simulink model "Sanepa_overall_model_Fault"  (R2023a)
settings: Solver=VariableStepAuto  StartTime=0.0  StopTime=5  RelTol=1e-3
undefined symbols (not defined in the file): D11, Delta
libraries: spsLoadFlowBusLib x44, spsThreePhaseTransformerTwoWindingsLib x23, spsThreePhaseParallelRLCLoadLib x23, spsThreePhasePISectionLineLib x18, spsThreePhaseVIMeasurementLib x4, spsThreePhaseFaultLib x4, spsThreePhaseSeriesRLCBranchLib x2, spspowerguiLib x1, spsThreePhaseSourceLib x1
settings Model: Creator=Isha Tiwari  LastModifiedBy=Dell
settings SolverCC: AlgebraicLoopSolver=TrustRegion
settings DataIOCC: SaveOutput=off  ReturnWorkspaceOutputs=off

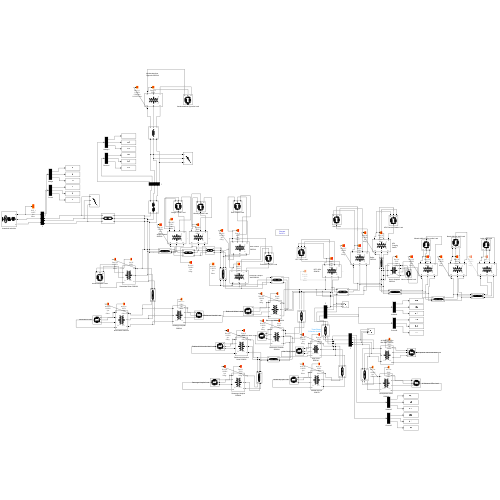
[thumbnail: Simulink's stored preview of the top-level diagram]
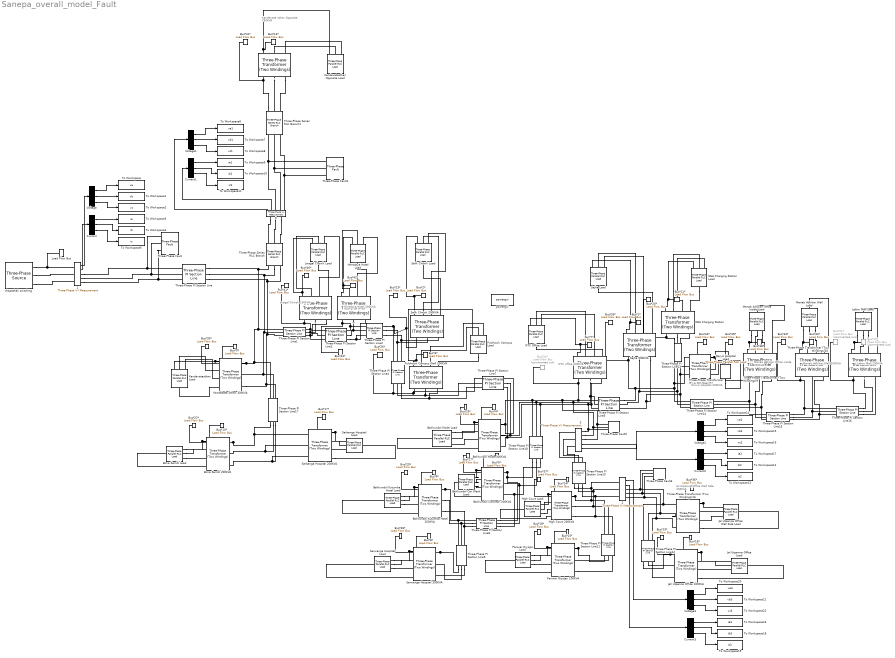
== system Sanepa_overall_model_Fault ==
  note: Norvic Hospital
      | 200KVA
  note: NTC office
      | 200KVA
  note: Manab Adhikar
      | Office inside
      | 200KVA
  note: Labim Mall
      | 200KVA
  note: Jal Utpanna Office
      | Wall Side 200KVA
  note: Manab Adhikar
      | Wall 200KVA
  note: Jwagal Chwok
      | 100KVA
  note: Himalaya Hotel
      | 300KVA
  note: Kandevata sthan
      | Opposite 250KVA
  . : spsThreePhaseTransformerTwoWindingsLib/Three-Phase Transformer (Two Windings)  Winding1Connection=Yg  Winding2Connection=Yg  CoreType=Three-limb core (core-type)  SetSaturation=off  Hysteresis=off  DataFile='hysteresis'  SetInitialFlux=off  Measurements=None  UNITS=pu  NominalPower=[ 500000 , 50 ]  Winding1=[11e3 , 0.002 , 0.08 ]  Winding2=[ 0.23e3 , 0.002 , 0.08 ]  Rm=500  Lm=500  L0=0.5  Saturation=[ 0,0 ; 0.0024,1.2 ; 1.0,1.52 ]  InitialFluxes=[ 0.8 , -0.8 , 0.7 ]  BreakLoop=off  DiscreteSolver=Trapezoidal iterative  DataType=off  TransfoNumber=1
  .. : spsThreePhaseTransformerTwoWindingsLib/Three-Phase Transformer (Two Windings)  Winding1Connection=Delta (D11)  Winding2Connection=Yn  CoreType=Three single-phase transformers  SetSaturation=off  Hysteresis=off  DataFile='hysteresis'  SetInitialFlux=off  Measurements=None  UNITS=pu  NominalPower=[ 200000 , 50 ]  Winding1=[ 11e3 , 0.002 , 0.08 ]  Winding2=[ 0.23e3 , 0.002 , 0.08 ]  Rm=500  Lm=500  L0=0.5  Saturation=[ 0,0 ; 0.0024,1.2 ; 1.0,1.52 ]  InitialFluxes=[ 0.8 , -0.8 , 0.7 ]  BreakLoop=off  DiscreteSolver=Trapezoidal iterative  DataType=off  TransfoNumber=1
  ... : spsThreePhaseTransformerTwoWindingsLib/Three-Phase Transformer (Two Windings)  Winding1Connection=Delta (D11)  Winding2Connection=Yn  CoreType=Three single-phase transformers  SetSaturation=off  Hysteresis=off  DataFile='hysteresis'  SetInitialFlux=off  Measurements=None  UNITS=pu  NominalPower=[ 200000 , 50 ]  Winding1=[11e3 , 0.002 , 0.08 ]  Winding2=[ 0.23e3 , 0.002 , 0.08 ]  Rm=500  Lm=500  L0=0.5  Saturation=[ 0,0 ; 0.0024,1.2 ; 1.0,1.52 ]  InitialFluxes=[ 0.8 , -0.8 , 0.7 ]  BreakLoop=off  DiscreteSolver=Trapezoidal iterative  DataType=off  TransfoNumber=1
  0 : spsThreePhaseVIMeasurementLib/Three-Phase V-I Measurement  VoltageMeasurement=phase-to-ground  SetLabelV=off  LabelV=V0  Vpu=on  VpuLL=off  CurrentMeasurement=yes  SetLabelI=off  LabelI=I634  Ipu=on  Pbase=100e6  Vbase=11000  OutputType=Magnitude  PhasorSimulation=off  PSBequivalent=0
  1 : spsThreePhaseVIMeasurementLib/Three-Phase V-I Measurement  VoltageMeasurement=phase-to-phase  SetLabelV=off  LabelV=V0  Vpu=on  VpuLL=off  CurrentMeasurement=yes  SetLabelI=off  LabelI=I634  Ipu=on  Pbase=100e6  Vbase=11000  OutputType=Magnitude  PhasorSimulation=off  PSBequivalent=0
  2 : spsThreePhaseVIMeasurementLib/Three-Phase V-I Measurement  VoltageMeasurement=phase-to-phase  SetLabelV=off  LabelV=V0  Vpu=on  VpuLL=off  CurrentMeasurement=yes  SetLabelI=off  LabelI=I634  Ipu=on  Pbase=100e6  Vbase=11000  OutputType=Magnitude  PhasorSimulation=off  PSBequivalent=0
  3 : spsThreePhaseVIMeasurementLib/Three-Phase V-I Measurement  VoltageMeasurement=phase-to-phase  SetLabelV=off  LabelV=V0  Vpu=on  VpuLL=off  CurrentMeasurement=yes  SetLabelI=off  LabelI=I634  Ipu=on  Pbase=100e6  Vbase=11000  OutputType=Magnitude  PhasorSimulation=off  PSBequivalent=0
  Bakhundol Car Wash Load : spsThreePhaseParallelRLCLoadLib/Three-Phase Parallel RLC Load  LConnTagsString=A|B|C  RConnTagsString=N  Configuration=Y (neutral)  NominalVoltage=230  Vabc=[1e3 1e3 1e3]  Vabcp=[1e3 1e3 1e3]  NominalFrequency=50  UnbalancedPower=off  ActivePower=25564.5  InductivePower=8402.643  CapacitivePower=0  Pabc=[22287 23379.5 18572.5]  QLabc=[7325.383 7684.47 6104.48]  QCabc=[0 0 0]  Pabcp=[10e3 9e3 11e3]  QLabcp=[100 90 110]  QCabcp=[100 90 110]  Measurements=None  LoadType=constant PQ
  Bakhundol Carwash 200KVA : spsThreePhaseTransformerTwoWindingsLib/Three-Phase Transformer (Two Windings)  Winding1Connection=Delta (D11)  Winding2Connection=Yn  CoreType=Three single-phase transformers  SetSaturation=off  Hysteresis=off  DataFile='hysteresis'  SetInitialFlux=off  Measurements=None  UNITS=pu  NominalPower=[ 200000 , 50 ]  Winding1=[ 11e3 , 0.002 , 0.08 ]  Winding2=[ 0.23e3 , 0.002 , 0.08 ]  Rm=500  Lm=500  L0=0.5  Saturation=[ 0,0 ; 0.0024,1.2 ; 1.0,1.52 ]  InitialFluxes=[ 0.8 , -0.8 , 0.7 ]  BreakLoop=off  DiscreteSolver=Trapezoidal iterative  DataType=off  TransfoNumber=1
  Bakhundol Kutumba Hotel 200KVA : spsThreePhaseTransformerTwoWindingsLib/Three-Phase Transformer (Two Windings)  Winding1Connection=Delta (D11)  Winding2Connection=Yn  CoreType=Three single-phase transformers  SetSaturation=off  Hysteresis=off  DataFile='hysteresis'  SetInitialFlux=off  Measurements=None  UNITS=pu  NominalPower=[ 200000 , 50 ]  Winding1=[ 11e3 , 0.002 , 0.08 ]  Winding2=[ 0.23e3 , 0.002 , 0.08 ]  Rm=500  Lm=500  L0=0.5  Saturation=[ 0,0 ; 0.0024,1.2 ; 1.0,1.52 ]  InitialFluxes=[ 0.8 , -0.8 , 0.7 ]  BreakLoop=off  DiscreteSolver=Trapezoidal iterative  DataType=off  TransfoNumber=1
  Bakhundol Kutumba Hotel Load : spsThreePhaseParallelRLCLoadLib/Three-Phase Parallel RLC Load  LConnTagsString=A|B|C  RConnTagsString=N  Configuration=Y (neutral)  NominalVoltage=230  Vabc=[1e3 1e3 1e3]  Vabcp=[1e3 1e3 1e3]  NominalFrequency=50  UnbalancedPower=off  ActivePower=15950.5  InductivePower=5242.672  CapacitivePower=0  Pabc=[22287 23379.5 18572.5]  QLabc=[7325.383 7684.47 6104.48]  QCabc=[0 0 0]  Pabcp=[10e3 9e3 11e3]  QLabcp=[100 90 110]  QCabcp=[100 90 110]  Measurements=None  LoadType=constant PQ
  Bakhundol Mode 300KVA : spsThreePhaseTransformerTwoWindingsLib/Three-Phase Transformer (Two Windings)  Winding1Connection=Delta (D11)  Winding2Connection=Yn  CoreType=Three single-phase transformers  SetSaturation=off  Hysteresis=off  DataFile='hysteresis'  SetInitialFlux=off  Measurements=None  UNITS=pu  NominalPower=[ 300000 , 50 ]  Winding1=[ 11e3 , 0.002 , 0.08 ]  Winding2=[ 0.23e3 , 0.002 , 0.08 ]  Rm=500  Lm=500  L0=0.5  Saturation=[ 0,0 ; 0.0024,1.2 ; 1.0,1.52 ]  InitialFluxes=[ 0.8 , -0.8 , 0.7 ]  BreakLoop=off  DiscreteSolver=Trapezoidal iterative  DataType=off  TransfoNumber=1
  Bakhundol Mode Load : spsThreePhaseParallelRLCLoadLib/Three-Phase Parallel RLC Load  LConnTagsString=A|B|C  RConnTagsString=N  Configuration=Y (neutral)  NominalVoltage=230  Vabc=[1e3 1e3 1e3]  Vabcp=[1e3 1e3 1e3]  NominalFrequency=50  UnbalancedPower=off  ActivePower=59640.5  InductivePower=19606.171  CapacitivePower=0  Pabc=[22287 23379.5 18572.5]  QLabc=[7325.383 7684.47 6104.48]  QCabc=[0 0 0]  Pabcp=[10e3 9e3 11e3]  QLabcp=[100 90 110]  QCabcp=[100 90 110]  Measurements=None  LoadType=constant PQ
  Bima Samiti 200KVA : spsThreePhaseTransformerTwoWindingsLib/Three-Phase Transformer (Two Windings)  Winding1Connection=Delta (D11)  Winding2Connection=Yn  CoreType=Three single-phase transformers  SetSaturation=off  Hysteresis=off  DataFile='hysteresis'  SetInitialFlux=off  Measurements=None  UNITS=pu  NominalPower=[ 200000 , 50 ]  Winding1=[ 11e3 , 0.002 , 0.08 ]  Winding2=[ 0.23e3 , 0.002 , 0.08 ]  Rm=500  Lm=500  L0=0.5  Saturation=[ 0,0 ; 0.0024,1.2 ; 1.0,1.52 ]  InitialFluxes=[ 0.8 , -0.8 , 0.7 ]  BreakLoop=off  DiscreteSolver=Trapezoidal iterative  DataType=off  TransfoNumber=1
  Bima Samiti Load : spsThreePhaseParallelRLCLoadLib/Three-Phase Parallel RLC Load  LConnTagsString=A|B|C  RConnTagsString=N  Configuration=Y (neutral)  NominalVoltage=230  Vabc=[1e3 1e3 1e3]  Vabcp=[1e3 1e3 1e3]  NominalFrequency=50  UnbalancedPower=off  ActivePower=30808.5  InductivePower=10126.263  CapacitivePower=0  Pabc=[22287 23379.5 18572.5]  QLabc=[7325.383 7684.47 6104.48]  QCabc=[0 0 0]  Pabcp=[10e3 9e3 11e3]  QLabcp=[100 90 110]  QCabcp=[100 90 110]  Measurements=None  LoadType=constant PQ
  Bus*1* : spsLoadFlowBusLib/Load Flow Bus  LConnTagsString=a  Phases=single  Connectors=on one side  ID=Bus*1*  Vbase=400  Vref=1  Vangle=0  VLF=1  VLFb=1  VLFc=1  angleLF=0  angleLFb=0  angleLFc=0
  Bus*10* : spsLoadFlowBusLib/Load Flow Bus  LConnTagsString=a  Phases=single  Connectors=on one side  ID=Bus*10*  Vbase=230  Vref=1  Vangle=0  VLF=1  VLFb=1  VLFc=1  angleLF=0  angleLFb=0  angleLFc=0
  Bus*11* : spsLoadFlowBusLib/Load Flow Bus  LConnTagsString=a  Phases=single  Connectors=on one side  ID=Bus*11*  Vbase=230  Vref=1  Vangle=0  VLF=1  VLFb=1  VLFc=1  angleLF=0  angleLFb=0  angleLFc=0
  Bus*12* : spsLoadFlowBusLib/Load Flow Bus  Commented=on  LConnTagsString=a  Phases=single  Connectors=on one side  ID=Bus*12*  Vbase=230  Vref=1  Vangle=0  VLF=1  VLFb=1  VLFc=1  angleLF=0  angleLFb=0  angleLFc=0
  Bus*13* : spsLoadFlowBusLib/Load Flow Bus  LConnTagsString=a  Phases=single  Connectors=on one side  ID=Bus*13*  Vbase=230  Vref=1  Vangle=0  VLF=0.9989  VLFb=1  VLFc=1  angleLF=-0.1488  angleLFb=0  angleLFc=0
  Bus*14* : spsLoadFlowBusLib/Load Flow Bus  LConnTagsString=a  Phases=single  Connectors=on one side  ID=Bus*14*  Vbase=230  Vref=1  Vangle=0  VLF=1  VLFb=1  VLFc=1  angleLF=0  angleLFb=0  angleLFc=0
  Bus*15* : spsLoadFlowBusLib/Load Flow Bus  LConnTagsString=a  Phases=single  Connectors=on one side  ID=Bus*15*  Vbase=230  Vref=1  Vangle=0  VLF=1  VLFb=1  VLFc=1  angleLF=0  angleLFb=0  angleLFc=0
  Bus*16* : spsLoadFlowBusLib/Load Flow Bus  LConnTagsString=a  Phases=single  Connectors=on one side  ID=Bus*16*  Vbase=230  Vref=1  Vangle=0  VLF=1  VLFb=1  VLFc=1  angleLF=0  angleLFb=0  angleLFc=0
  Bus*17* : spsLoadFlowBusLib/Load Flow Bus  LConnTagsString=a  Phases=single  Connectors=on one side  ID=Bus*17*  Vbase=230  Vref=1  Vangle=0  VLF=1  VLFb=1  VLFc=1  angleLF=0  angleLFb=0  angleLFc=0
  Bus*18* : spsLoadFlowBusLib/Load Flow Bus  LConnTagsString=a  Phases=single  Connectors=on one side  ID=Bus*18*  Vbase=11000  Vref=1  Vangle=0  VLF=1  VLFb=1  VLFc=1  angleLF=0  angleLFb=0  angleLFc=0
  Bus*19* : spsLoadFlowBusLib/Load Flow Bus  LConnTagsString=a  Phases=single  Connectors=on one side  ID=Bus*19*  Vbase=11000  Vref=1  Vangle=0  VLF=1  VLFb=1  VLFc=1  angleLF=0  angleLFb=0  angleLFc=0
  Bus*2* : spsLoadFlowBusLib/Load Flow Bus  LConnTagsString=a  Phases=single  Connectors=on one side  ID=Bus*2*  Vbase=230  Vref=1  Vangle=0  VLF=1  VLFb=1  VLFc=1  angleLF=0  angleLFb=0  angleLFc=0
  Bus*20* : spsLoadFlowBusLib/Load Flow Bus  LConnTagsString=a  Phases=single  Connectors=on one side  ID=Bus*20*  Vbase=11000  Vref=1  Vangle=0  VLF=1  VLFb=1  VLFc=1  angleLF=0  angleLFb=0  angleLFc=0
  Bus*21* : spsLoadFlowBusLib/Load Flow Bus  Commented=on  LConnTagsString=a  Phases=single  Connectors=on one side  ID=Bus*21*  Vbase=11000  Vref=1  Vangle=0  VLF=1  VLFb=1  VLFc=1  angleLF=0  angleLFb=0  angleLFc=0
  Bus*22* : spsLoadFlowBusLib/Load Flow Bus  LConnTagsString=a  Phases=single  Connectors=on one side  ID=Bus*22*  Vbase=11000  Vref=1  Vangle=0  VLF=1  VLFb=1  VLFc=1  angleLF=0  angleLFb=0  angleLFc=0
  Bus*23* : spsLoadFlowBusLib/Load Flow Bus  LConnTagsString=a  Phases=single  Connectors=on one side  ID=Bus*23*  Vbase=11000  Vref=1  Vangle=0  VLF=1  VLFb=1  VLFc=1  angleLF=0  angleLFb=0  angleLFc=0
  Bus*24* : spsLoadFlowBusLib/Load Flow Bus  Commented=on  LConnTagsString=a  Phases=single  Connectors=on one side  ID=Bus*24*  Vbase=11000  Vref=1  Vangle=0  VLF=1  VLFb=1  VLFc=1  angleLF=0  angleLFb=0  angleLFc=0
  Bus*25* : spsLoadFlowBusLib/Load Flow Bus  LConnTagsString=a  Phases=single  Connectors=on one side  ID=Bus*25*  Vbase=11000  Vref=1  Vangle=0  VLF=1  VLFb=1  VLFc=1  angleLF=0  angleLFb=0  angleLFc=0
  Bus*26* : spsLoadFlowBusLib/Load Flow Bus  LConnTagsString=a  Phases=single  Connectors=on one side  ID=Bus*26*  Vbase=11000  Vref=1  Vangle=0  VLF=1  VLFb=1  VLFc=1  angleLF=0  angleLFb=0  angleLFc=0
  Bus*27* : spsLoadFlowBusLib/Load Flow Bus  LConnTagsString=a  Phases=single  Connectors=on one side  ID=Bus*27*  Vbase=11000  Vref=1  Vangle=0  VLF=1  VLFb=1  VLFc=1  angleLF=0  angleLFb=0  angleLFc=0
  Bus*28* : spsLoadFlowBusLib/Load Flow Bus  LConnTagsString=a  Phases=single  Connectors=on one side  ID=Bus*28*  Vbase=11000  Vref=1  Vangle=0  VLF=1  VLFb=1  VLFc=1  angleLF=0  angleLFb=0  angleLFc=0
  Bus*29* : spsLoadFlowBusLib/Load Flow Bus  LConnTagsString=a  Phases=single  Connectors=on one side  ID=Bus*29*  Vbase=11000  Vref=1  Vangle=0  VLF=1  VLFb=1  VLFc=1  angleLF=0  angleLFb=0  angleLFc=0
  Bus*3* : spsLoadFlowBusLib/Load Flow Bus  LConnTagsString=a  Phases=single  Connectors=on one side  ID=Bus*3*  Vbase=230  Vref=1  Vangle=0  VLF=1  VLFb=1  VLFc=1  angleLF=0  angleLFb=0  angleLFc=0
  Bus*30* : spsLoadFlowBusLib/Load Flow Bus  LConnTagsString=a  Phases=single  Connectors=on one side  ID=Bus*30*  Vbase=11000  Vref=1  Vangle=0  VLF=1  VLFb=1  VLFc=1  angleLF=0  angleLFb=0  angleLFc=0
  Bus*31* : spsLoadFlowBusLib/Load Flow Bus  LConnTagsString=a  Phases=single  Connectors=on one side  ID=Bus*31*  Vbase=11000  Vref=1  Vangle=0  VLF=0.9999  VLFb=1  VLFc=1  angleLF=-0.004876  angleLFb=0  angleLFc=0
  Bus*32* : spsLoadFlowBusLib/Load Flow Bus  LConnTagsString=a  Phases=single  Connectors=on one side  ID=Bus*32*  Vbase=230  Vref=1  Vangle=0  VLF=1  VLFb=1  VLFc=1  angleLF=0  angleLFb=0  angleLFc=0
  Bus*33* : spsLoadFlowBusLib/Load Flow Bus  LConnTagsString=a  Phases=single  Connectors=on one side  ID=Bus*33*  Vbase=11000  Vref=1  Vangle=0  VLF=1  VLFb=1  VLFc=1  angleLF=0  angleLFb=0  angleLFc=0
  Bus*34* : spsLoadFlowBusLib/Load Flow Bus  LConnTagsString=a  Phases=single  Connectors=on one side  ID=Bus*34*  Vbase=230  Vref=1  Vangle=0  VLF=1  VLFb=1  VLFc=1  angleLF=0  angleLFb=0  angleLFc=0
  Bus*35* : spsLoadFlowBusLib/Load Flow Bus  LConnTagsString=a  Phases=single  Connectors=on one side  ID=Bus*35*  Vbase=11000  Vref=1  Vangle=0  VLF=1  VLFb=1  VLFc=1  angleLF=0  angleLFb=0  angleLFc=0
  Bus*36* : spsLoadFlowBusLib/Load Flow Bus  LConnTagsString=a  Phases=single  Connectors=on one side  ID=Bus*36*  Vbase=230  Vref=1  Vangle=0  VLF=1  VLFb=1  VLFc=1  angleLF=0  angleLFb=0  angleLFc=0
  Bus*37* : spsLoadFlowBusLib/Load Flow Bus  LConnTagsString=a  Phases=single  Connectors=on one side  ID=Bus*37*  Vbase=11000  Vref=1  Vangle=0  VLF=1  VLFb=1  VLFc=1  angleLF=0  angleLFb=0  angleLFc=0
  Bus*38* : spsLoadFlowBusLib/Load Flow Bus  LConnTagsString=a  Phases=single  Connectors=on one side  ID=Bus*38*  Vbase=230  Vref=1  Vangle=0  VLF=1  VLFb=1  VLFc=1  angleLF=0  angleLFb=0  angleLFc=0
  Bus*39* : spsLoadFlowBusLib/Load Flow Bus  LConnTagsString=a  Phases=single  Connectors=on one side  ID=Bus*39*  Vbase=11000  Vref=1  Vangle=0  VLF=1  VLFb=1  VLFc=1  angleLF=0  angleLFb=0  angleLFc=0
  Bus*4* : spsLoadFlowBusLib/Load Flow Bus  LConnTagsString=a  Phases=single  Connectors=on one side  ID=Bus*4*  Vbase=230  Vref=1  Vangle=0  VLF=1  VLFb=1  VLFc=1  angleLF=0  angleLFb=0  angleLFc=0
  Bus*40* : spsLoadFlowBusLib/Load Flow Bus  LConnTagsString=a  Phases=single  Connectors=on one side  ID=Bus*40*  Vbase=230  Vref=1  Vangle=0  VLF=1  VLFb=1  VLFc=1  angleLF=0  angleLFb=0  angleLFc=0
  Bus*41* : spsLoadFlowBusLib/Load Flow Bus  LConnTagsString=a  Phases=single  Connectors=on one side  ID=Bus*41*  Vbase=11000  Vref=1  Vangle=0  VLF=1  VLFb=1  VLFc=1  angleLF=0  angleLFb=0  angleLFc=0
  Bus*42* : spsLoadFlowBusLib/Load Flow Bus  LConnTagsString=a  Phases=single  Connectors=on one side  ID=Bus*42*  Vbase=230  Vref=1  Vangle=0  VLF=1  VLFb=1  VLFc=1  angleLF=0  angleLFb=0  angleLFc=0
  Bus*43* : spsLoadFlowBusLib/Load Flow Bus  LConnTagsString=a  Phases=single  Connectors=on one side  ID=Bus*43*  Vbase=11000  Vref=1  Vangle=0  VLF=1  VLFb=1  VLFc=1  angleLF=0  angleLFb=0  angleLFc=0
  Bus*5* : spsLoadFlowBusLib/Load Flow Bus  LConnTagsString=a  Phases=single  Connectors=on one side  ID=Bus*5*  Vbase=230  Vref=1  Vangle=0  VLF=1  VLFb=1  VLFc=1  angleLF=0  angleLFb=0  angleLFc=0
  Bus*6* : spsLoadFlowBusLib/Load Flow Bus  LConnTagsString=a  Phases=single  Connectors=on one side  ID=Bus*6*  Vbase=230  Vref=1  Vangle=0  VLF=1  VLFb=1  VLFc=1  angleLF=0  angleLFb=0  angleLFc=0
  Bus*7* : spsLoadFlowBusLib/Load Flow Bus  LConnTagsString=a  Phases=single  Connectors=on one side  ID=Bus*7*  Vbase=230  Vref=1  Vangle=0  VLF=1  VLFb=1  VLFc=1  angleLF=0  angleLFb=0  angleLFc=0
  Bus*8* : spsLoadFlowBusLib/Load Flow Bus  LConnTagsString=a  Phases=single  Connectors=on one side  ID=Bus*8*  Vbase=230  Vref=1  Vangle=0  VLF=1  VLFb=1  VLFc=1  angleLF=0  angleLFb=0  angleLFc=0
  Bus*9* : spsLoadFlowBusLib/Load Flow Bus  LConnTagsString=a  Phases=single  Connectors=on one side  ID=Bus*9*  Vbase=230  Vref=1  Vangle=0  VLF=1  VLFb=1  VLFc=1  angleLF=0  angleLFb=0  angleLFc=0
  Current{,1..3} (4 alike) : Demux  Outputs=3
  HIgh Court Load : spsThreePhaseParallelRLCLoadLib/Three-Phase Parallel RLC Load  LConnTagsString=A|B|C  RConnTagsString=N  Configuration=Y (neutral)  NominalVoltage=230  Vabc=[1e3 1e3 1e3]  Vabcp=[1e3 1e3 1e3]  NominalFrequency=50  UnbalancedPower=off  ActivePower=12017.5  InductivePower=3904.961  CapacitivePower=0  Pabc=[22287 23379.5 18572.5]  QLabc=[7325.383 7684.47 6104.48]  QCabc=[0 0 0]  Pabcp=[10e3 9e3 11e3]  QLabcp=[100 90 110]  QCabcp=[100 90 110]  Measurements=None  LoadType=constant PQ
  HImalaya Hotel Load : spsThreePhaseParallelRLCLoadLib/Three-Phase Parallel RLC Load  LConnTagsString=A|B|C  RConnTagsString=N  Configuration=Y (neutral)  NominalVoltage=230  Vabc=[1e3 1e3 1e3]  Vabcp=[1e3 1e3 1e3]  NominalFrequency=50  UnbalancedPower=off  ActivePower=29497.5  InductivePower=9695.359  CapacitivePower=0  Pabc=[22287 23379.5 18572.5]  QLabc=[7325.383 7684.47 6104.48]  QCabc=[0 0 0]  Pabcp=[10e3 9e3 11e3]  QLabcp=[100 90 110]  QCabcp=[100 90 110]  Measurements=None  LoadType=constant PQ
  High Court 200KVA : spsThreePhaseTransformerTwoWindingsLib/Three-Phase Transformer (Two Windings)  Winding1Connection=Delta (D11)  Winding2Connection=Yn  CoreType=Three single-phase transformers  SetSaturation=off  Hysteresis=off  DataFile='hysteresis'  SetInitialFlux=off  Measurements=None  UNITS=pu  NominalPower=[ 200000 , 50 ]  Winding1=[ 11e3 , 0.002 , 0.08 ]  Winding2=[ 0.23e3 , 0.002 , 0.08 ]  Rm=500  Lm=500  L0=0.5  Saturation=[ 0,0 ; 0.0024,1.2 ; 1.0,1.52 ]  InitialFluxes=[ 0.8 , -0.8 , 0.7 ]  BreakLoop=off  DiscreteSolver=Trapezoidal iterative  DataType=off  TransfoNumber=1
  Jal Utpanna Office Load : spsThreePhaseParallelRLCLoadLib/Three-Phase Parallel RLC Load  LConnTagsString=A|B|C  RConnTagsString=N  Configuration=Y (neutral)  NominalVoltage=230  Vabc=[1e3 1e3 1e3]  Vabcp=[1e3 1e3 1e3]  NominalFrequency=50  UnbalancedPower=off  ActivePower=34741.5  InductivePower=11418.978  CapacitivePower=0  Pabc=[22287 23379.5 18572.5]  QLabc=[7325.383 7684.47 6104.48]  QCabc=[0 0 0]  Pabcp=[10e3 9e3 11e3]  QLabcp=[100 90 110]  QCabcp=[100 90 110]  Measurements=None  LoadType=constant PQ
  Jal Utpanna Office Wall Side Load : spsThreePhaseParallelRLCLoadLib/Three-Phase Parallel RLC Load  LConnTagsString=A|B|C  RConnTagsString=N  Configuration=Y (neutral)  NominalVoltage=230  Vabc=[1e3 1e3 1e3]  Vabcp=[1e3 1e3 1e3]  NominalFrequency=50  UnbalancedPower=off  ActivePower=34741.5  InductivePower=11418.978  CapacitivePower=0  Pabc=[22287 23379.5 18572.5]  QLabc=[7325.383 7684.47 6104.48]  QCabc=[0 0 0]  Pabcp=[10e3 9e3 11e3]  QLabcp=[100 90 110]  QCabcp=[100 90 110]  Measurements=None  LoadType=constant PQ
  Jall Utpanna Office 100KVA : spsThreePhaseTransformerTwoWindingsLib/Three-Phase Transformer (Two Windings)  Winding1Connection=Delta (D11)  Winding2Connection=Yn  CoreType=Three single-phase transformers  SetSaturation=off  Hysteresis=off  DataFile='hysteresis'  SetInitialFlux=off  Measurements=None  UNITS=pu  NominalPower=[ 100000 , 50 ]  Winding1=[ 11e3 , 0.002 , 0.08 ]  Winding2=[ 0.23e3 , 0.002 , 0.08 ]  Rm=500  Lm=500  L0=0.5  Saturation=[ 0,0 ; 0.0024,1.2 ; 1.0,1.52 ]  InitialFluxes=[ 0.8 , -0.8 , 0.7 ]  BreakLoop=off  DiscreteSolver=Trapezoidal iterative  DataType=off  TransfoNumber=1
  Jwagal Chowk Load : spsThreePhaseParallelRLCLoadLib/Three-Phase Parallel RLC Load  LConnTagsString=A|B|C  RConnTagsString=N  Configuration=Y (neutral)  NominalVoltage=230  Vabc=[1e3 1e3 1e3]  Vabcp=[1e3 1e3 1e3]  NominalFrequency=50  UnbalancedPower=off  ActivePower=21850  InductivePower=7181.748  CapacitivePower=0  Pabc=[22287 23379.5 18572.5]  QLabc=[7325.383 7684.47 6104.48]  QCabc=[0 0 0]  Pabcp=[10e3 9e3 11e3]  QLabcp=[100 90 110]  QCabcp=[100 90 110]  Measurements=None  LoadType=constant PQ
  Kandebata Sthan 300KVA : spsThreePhaseTransformerTwoWindingsLib/Three-Phase Transformer (Two Windings)  Winding1Connection=Delta (D11)  Winding2Connection=Yn  CoreType=Three single-phase transformers  SetSaturation=off  Hysteresis=off  DataFile='hysteresis'  SetInitialFlux=off  Measurements=None  UNITS=pu  NominalPower=[ 300000 , 50 ]  Winding1=[ 11e3 , 0.002 , 0.08 ]  Winding2=[ 0.23e3 , 0.002 , 0.08 ]  Rm=500  Lm=500  L0=0.5  Saturation=[ 0,0 ; 0.0024,1.2 ; 1.0,1.52 ]  InitialFluxes=[ 0.8 , -0.8 , 0.7 ]  BreakLoop=off  DiscreteSolver=Trapezoidal iterative  DataType=off  TransfoNumber=1
  Kandevatasthan Load : spsThreePhaseParallelRLCLoadLib/Three-Phase Parallel RLC Load  LConnTagsString=A|B|C  RConnTagsString=N  Configuration=Y (neutral)  NominalVoltage=230  Vabc=[1e3 1e3 1e3]  Vabcp=[1e3 1e3 1e3]  NominalFrequency=50  UnbalancedPower=off  ActivePower=68827.5  InductivePower=22622.506  CapacitivePower=0  Pabc=[22287 23379.5 18572.5]  QLabc=[7325.383 7684.47 6104.48]  QCabc=[0 0 0]  Pabcp=[10e3 9e3 11e3]  QLabcp=[100 90 110]  QCabcp=[100 90 110]  Measurements=None  LoadType=constant PQ
  Kandevatasthan Opposite Load : spsThreePhaseParallelRLCLoadLib/Three-Phase Parallel RLC Load  LConnTagsString=A|B|C  Configuration=Y (grounded)  NominalVoltage=230  Vabc=[1e3 1e3 1e3]  Vabcp=[1e3 1e3 1e3]  NominalFrequency=50  UnbalancedPower=off  ActivePower=64239  InductivePower=21114.33  CapacitivePower=0  Pabc=[22287 23379.5 18572.5]  QLabc=[7325.383 7684.47 6104.48]  QCabc=[0 0 0]  Pabcp=[10e3 9e3 11e3]  QLabcp=[100 90 110]  QCabcp=[100 90 110]  Measurements=None  LoadType=constant PQ
  Labim Mall Load : spsThreePhaseParallelRLCLoadLib/Three-Phase Parallel RLC Load  LConnTagsString=A|B|C  RConnTagsString=N  Configuration=Y (neutral)  NominalVoltage=230  Vabc=[1e3 1e3 1e3]  Vabcp=[1e3 1e3 1e3]  NominalFrequency=50  UnbalancedPower=off  ActivePower=28500  InductivePower=9367.5  CapacitivePower=0  Pabc=[22287 23379.5 18572.5]  QLabc=[7325.383 7684.47 6104.48]  QCabc=[0 0 0]  Pabcp=[10e3 9e3 11e3]  QLabcp=[100 90 110]  QCabcp=[100 90 110]  Measurements=None  LoadType=constant PQ
  Load Flow Bus : spsLoadFlowBusLib/Load Flow Bus  LConnTagsString=a  Phases=single  Connectors=on one side  ID=BUS_1  Vbase=11e3  Vref=1  Vangle=0  VLF=1  VLFb=1  VLFc=1  angleLF=0  angleLFb=0  angleLFc=0
  Manab Adhikar Office Inside Load : spsThreePhaseParallelRLCLoadLib/Three-Phase Parallel RLC Load  LConnTagsString=A|B|C  RConnTagsString=N  Configuration=Y (neutral)  NominalVoltage=230  Vabc=[1e3 1e3 1e3]  Vabcp=[1e3 1e3 1e3]  NominalFrequency=50  UnbalancedPower=off  ActivePower=28500  InductivePower=9367.5  CapacitivePower=0  Pabc=[22287 23379.5 18572.5]  QLabc=[7325.383 7684.47 6104.48]  QCabc=[0 0 0]  Pabcp=[10e3 9e3 11e3]  QLabcp=[100 90 110]  QCabcp=[100 90 110]  Measurements=None  LoadType=constant PQ
  Manab Adhikar Wall Load : spsThreePhaseParallelRLCLoadLib/Three-Phase Parallel RLC Load  LConnTagsString=A|B|C  RConnTagsString=N  Configuration=Y (neutral)  NominalVoltage=230  Vabc=[1e3 1e3 1e3]  Vabcp=[1e3 1e3 1e3]  NominalFrequency=50  UnbalancedPower=off  ActivePower=28500  InductivePower=9367.5  CapacitivePower=0  Pabc=[22287 23379.5 18572.5]  QLabc=[7325.383 7684.47 6104.48]  QCabc=[0 0 0]  Pabcp=[10e3 9e3 11e3]  QLabcp=[100 90 110]  QCabcp=[100 90 110]  Measurements=None  LoadType=constant PQ
  NEA Charging Station : spsThreePhaseTransformerTwoWindingsLib/Three-Phase Transformer (Two Windings)  Winding1Connection=Delta (D11)  Winding2Connection=Yn  CoreType=Three single-phase transformers  SetSaturation=off  Hysteresis=off  DataFile='hysteresis'  SetInitialFlux=off  Measurements=None  UNITS=pu  NominalPower=[ 200000 , 50 ]  Winding1=[ 11e3 , 0.002 , 0.08 ]  Winding2=[ 0.23e3 , 0.002 , 0.08 ]  Rm=500  Lm=500  L0=0.5  Saturation=[ 0,0 ; 0.0024,1.2 ; 1.0,1.52 ]  InitialFluxes=[ 0.8 , -0.8 , 0.7 ]  BreakLoop=off  DiscreteSolver=Trapezoidal iterative  DataType=off  TransfoNumber=1
  NEA Charging Station Load : spsThreePhaseParallelRLCLoadLib/Three-Phase Parallel RLC Load  LConnTagsString=A|B|C  RConnTagsString=N  Configuration=Y (neutral)  NominalVoltage=230  Vabc=[1e3 1e3 1e3]  Vabcp=[1e3 1e3 1e3]  NominalFrequency=50  UnbalancedPower=off  ActivePower=28500  InductivePower=9367.5  CapacitivePower=0  Pabc=[22287 23379.5 18572.5]  QLabc=[7325.383 7684.47 6104.48]  QCabc=[0 0 0]  Pabcp=[10e3 9e3 11e3]  QLabcp=[100 90 110]  QCabcp=[100 90 110]  Measurements=None  LoadType=constant PQ
  NTC Office Load : spsThreePhaseParallelRLCLoadLib/Three-Phase Parallel RLC Load  LConnTagsString=A|B|C  RConnTagsString=N  Configuration=Y (neutral)  NominalVoltage=230  Vabc=[1e3 1e3 1e3]  Vabcp=[1e3 1e3 1e3]  NominalFrequency=50  UnbalancedPower=off  ActivePower=68827.5  InductivePower=22622.497  CapacitivePower=0  Pabc=[22287 23379.5 18572.5]  QLabc=[7325.383 7684.47 6104.48]  QCabc=[0 0 0]  Pabcp=[10e3 9e3 11e3]  QLabcp=[100 90 110]  QCabcp=[100 90 110]  Measurements=None  LoadType=constant PQ
  Norvic Hospital Load : spsThreePhaseParallelRLCLoadLib/Three-Phase Parallel RLC Load  LConnTagsString=A|B|C  RConnTagsString=N  Configuration=Y (neutral)  NominalVoltage=230  Vabc=[1e3 1e3 1e3]  Vabcp=[1e3 1e3 1e3]  NominalFrequency=50  UnbalancedPower=off  ActivePower=28500  InductivePower=9367.5  CapacitivePower=0  Pabc=[22287 23379.5 18572.5]  QLabc=[7325.383 7684.47 6104.48]  QCabc=[0 0 0]  Pabcp=[10e3 9e3 11e3]  QLabcp=[100 90 110]  QCabcp=[100 90 110]  Measurements=None  LoadType=constant PQ
  Pariwar Niyojan 100KVA : spsThreePhaseTransformerTwoWindingsLib/Three-Phase Transformer (Two Windings)  Winding1Connection=Delta (D11)  Winding2Connection=Yn  CoreType=Three single-phase transformers  SetSaturation=off  Hysteresis=off  DataFile='hysteresis'  SetInitialFlux=off  Measurements=None  UNITS=pu  NominalPower=[ 100000 , 50 ]  Winding1=[ 11e3 , 0.002 , 0.08 ]  Winding2=[ 0.23e3 , 0.002 , 0.08 ]  Rm=500  Lm=500  L0=0.5  Saturation=[ 0,0 ; 0.0024,1.2 ; 1.0,1.52 ]  InitialFluxes=[ 0.8 , -0.8 , 0.7 ]  BreakLoop=off  DiscreteSolver=Trapezoidal iterative  DataType=off  TransfoNumber=1
  Pariwar Niyojan Load : spsThreePhaseParallelRLCLoadLib/Three-Phase Parallel RLC Load  LConnTagsString=A|B|C  RConnTagsString=N  Configuration=Y (neutral)  NominalVoltage=230  Vabc=[1e3 1e3 1e3]  Vabcp=[1e3 1e3 1e3]  NominalFrequency=50  UnbalancedPower=off  ActivePower=10988  InductivePower=3447.231  CapacitivePower=0  Pabc=[22287 23379.5 18572.5]  QLabc=[7325.383 7684.47 6104.48]  QCabc=[0 0 0]  Pabcp=[10e3 9e3 11e3]  QLabcp=[100 90 110]  QCabcp=[100 90 110]  Measurements=None  LoadType=constant PQ
  Pulchowk Campus Load : spsThreePhaseParallelRLCLoadLib/Three-Phase Parallel RLC Load  LConnTagsString=A|B|C  RConnTagsString=N  Configuration=Y (neutral)  NominalVoltage=230  Vabc=[1e3 1e3 1e3]  Vabcp=[1e3 1e3 1e3]  NominalFrequency=50  UnbalancedPower=off  ActivePower=38019.33  InductivePower=12496.241  CapacitivePower=0  Pabc=[22287 23379.5 18572.5]  QLabc=[7325.383 7684.47 6104.48]  QCabc=[0 0 0]  Pabcp=[10e3 9e3 11e3]  QLabcp=[100 90 110]  QCabcp=[100 90 110]  Measurements=None  LoadType=constant PQ
  Pulchwok Campus Wall 200KVA : spsThreePhaseTransformerTwoWindingsLib/Three-Phase Transformer (Two Windings)  Winding1Connection=Delta (D11)  Winding2Connection=Yn  CoreType=Three single-phase transformers  SetSaturation=off  Hysteresis=off  DataFile='hysteresis'  SetInitialFlux=off  Measurements=None  UNITS=pu  NominalPower=[ 100000 , 50 ]  Winding1=[ 11e3 , 0.002 , 0.08 ]  Winding2=[ 0.23e3 , 0.002 , 0.08 ]  Rm=500  Lm=500  L0=0.5  Saturation=[ 0,0 ; 0.0024,1.2 ; 1.0,1.52 ]  InitialFluxes=[ 0.8 , -0.8 , 0.7 ]  BreakLoop=off  DiscreteSolver=Trapezoidal iterative  DataType=off  TransfoNumber=1
  Sajha 500KVA : spsThreePhaseTransformerTwoWindingsLib/Three-Phase Transformer (Two Windings)  Winding1Connection=Delta (D11)  Winding2Connection=Yn  CoreType=Three single-phase transformers  SetSaturation=off  Hysteresis=off  DataFile='hysteresis'  SetInitialFlux=off  Measurements=None  UNITS=pu  NominalPower=[ 500000 , 50 ]  Winding1=[ 11e3 , 0.002 , 0.08 ]  Winding2=[ 0.40e3 , 0.002 , 0.08 ]  Rm=500  Lm=500  L0=0.5  Saturation=[ 0,0 ; 0.0024,1.2 ; 1.0,1.52 ]  InitialFluxes=[ 0.8 , -0.8 , 0.7 ]  BreakLoop=off  DiscreteSolver=Trapezoidal iterative  DataType=off  TransfoNumber=1
  Sajha Load : spsThreePhaseParallelRLCLoadLib/Three-Phase Parallel RLC Load  LConnTagsString=A|B|C  RConnTagsString=N  Configuration=Y (neutral)  NominalVoltage=230  Vabc=[1e3 1e3 1e3]  Vabcp=[1e3 1e3 1e3]  NominalFrequency=50  UnbalancedPower=off  ActivePower=68827.5  InductivePower=22622.497  CapacitivePower=0  Pabc=[22287 23379.5 18572.5]  QLabc=[7325.383 7684.47 6104.48]  QCabc=[0 0 0]  Pabcp=[10e3 9e3 11e3]  QLabcp=[100 90 110]  QCabcp=[100 90 110]  Measurements=None  LoadType=constant PQ
  Salik Chowk Load : spsThreePhaseParallelRLCLoadLib/Three-Phase Parallel RLC Load  LConnTagsString=A|B|C  RConnTagsString=N  Configuration=Y (neutral)  NominalVoltage=230  Vabc=[1e3 1e3 1e3]  Vabcp=[1e3 1e3 1e3]  NominalFrequency=50  UnbalancedPower=off  ActivePower=19883.5  InductivePower=6535.388  CapacitivePower=0  Pabc=[22287 23379.5 18572.5]  QLabc=[7325.383 7684.47 6104.48]  QCabc=[0 0 0]  Pabcp=[10e3 9e3 11e3]  QLabcp=[100 90 110]  QCabcp=[100 90 110]  Measurements=None  LoadType=constant PQ
  Salik Chwok 200KVA : spsThreePhaseTransformerTwoWindingsLib/Three-Phase Transformer (Two Windings)  Winding1Connection=Delta (D11)  Winding2Connection=Yn  CoreType=Three single-phase transformers  SetSaturation=off  Hysteresis=off  DataFile='hysteresis'  SetInitialFlux=off  Measurements=None  UNITS=pu  NominalPower=[ 200000 , 50 ]  Winding1=[11e3 , 0.002 , 0.08 ]  Winding2=[ 0.23e3 , 0.002 , 0.08 ]  Rm=500  Lm=500  L0=0.5  Saturation=[ 0,0 ; 0.0024,1.2 ; 1.0,1.52 ]  InitialFluxes=[ 0.8 , -0.8 , 0.7 ]  BreakLoop=off  DiscreteSolver=Trapezoidal iterative  DataType=off  TransfoNumber=1
  Sarbanga Hospital 200KVA : spsThreePhaseTransformerTwoWindingsLib/Three-Phase Transformer (Two Windings)  Winding1Connection=Delta (D11)  Winding2Connection=Yn  CoreType=Three single-phase transformers  SetSaturation=off  Hysteresis=off  DataFile='hysteresis'  SetInitialFlux=off  Measurements=None  UNITS=pu  NominalPower=[ 200000 , 50 ]  Winding1=[ 11e3 , 0.002 , 0.08 ]  Winding2=[ 0.23e3 , 0.002 , 0.08 ]  Rm=500  Lm=500  L0=0.5  Saturation=[ 0,0 ; 0.0024,1.2 ; 1.0,1.52 ]  InitialFluxes=[ 0.8 , -0.8 , 0.7 ]  BreakLoop=off  DiscreteSolver=Trapezoidal iterative  DataType=off  TransfoNumber=1
  Sarbanga Hospital Load : spsThreePhaseParallelRLCLoadLib/Three-Phase Parallel RLC Load  LConnTagsString=A|B|C  RConnTagsString=N  Configuration=Y (neutral)  NominalVoltage=230  Vabc=[1e3 1e3 1e3]  Vabcp=[1e3 1e3 1e3]  NominalFrequency=50  UnbalancedPower=off  ActivePower=46682  InductivePower=15225.305  CapacitivePower=0  Pabc=[22287 23379.5 18572.5]  QLabc=[7325.383 7684.47 6104.48]  QCabc=[0 0 0]  Pabcp=[10e3 9e3 11e3]  QLabcp=[100 90 110]  QCabcp=[100 90 110]  Measurements=None  LoadType=constant PQ
  Sarwanga Hospital 300KVA : spsThreePhaseTransformerTwoWindingsLib/Three-Phase Transformer (Two Windings)  Winding1Connection=Delta (D11)  Winding2Connection=Yn  CoreType=Three single-phase transformers  SetSaturation=off  Hysteresis=off  DataFile='hysteresis'  SetInitialFlux=off  Measurements=None  UNITS=pu  NominalPower=[ 300000 , 50 ]  Winding1=[ 11e3 , 0.002 , 0.08 ]  Winding2=[ 0.23e3 , 0.002 , 0.08 ]  Rm=500  Lm=500  L0=0.5  Saturation=[ 0,0 ; 0.0024,1.2 ; 1.0,1.52 ]  InitialFluxes=[ 0.8 , -0.8 , 0.7 ]  BreakLoop=off  DiscreteSolver=Trapezoidal iterative  DataType=off  TransfoNumber=1
  Sarwanga Hospital Load : spsThreePhaseParallelRLCLoadLib/Three-Phase Parallel RLC Load  LConnTagsString=A|B|C  RConnTagsString=N  Configuration=Y (neutral)  NominalVoltage=230  Vabc=[1e3 1e3 1e3]  Vabcp=[1e3 1e3 1e3]  NominalFrequency=50  UnbalancedPower=off  ActivePower=51373.5  InductivePower=16589.837  CapacitivePower=0  Pabc=[22287 23379.5 18572.5]  QLabc=[7325.383 7684.47 6104.48]  QCabc=[0 0 0]  Pabcp=[10e3 9e3 11e3]  QLabcp=[100 90 110]  QCabcp=[100 90 110]  Measurements=None  LoadType=constant PQ
  Three-Phase PI Section Line : spsThreePhasePISectionLineLib/Three-Phase PI Section Line  LConnTagsString=a|b|c  RConnTagsString=A|B|C  Length=0.225  Frequency=50  Resistances=[ 0.01273 0.3864]  Inductances="[ 0.9337e-3  4.1264e-3]"  Capacitances=[12.74e-9 7.751e-9]
  Three-Phase PI Section Line1 : spsThreePhasePISectionLineLib/Three-Phase PI Section Line  LConnTagsString=a|b|c  RConnTagsString=A|B|C  Length=0.25  Frequency=50  Resistances=[ 0.01273 0.3864]  Inductances="[ 0.9337e-3  4.1264e-3]"  Capacitances=[12.74e-9 7.751e-9]
  Three-Phase PI Section Line{2..5,7..18} (16 alike) : spsThreePhasePISectionLineLib/Three-Phase PI Section Line  LConnTagsString=a|b|c  RConnTagsString=A|B|C  Length=0.3  Frequency=50  Resistances=[ 0.01273 0.3864]  Inductances="[ 0.9337e-3  4.1264e-3]"  Capacitances=[12.74e-9 7.751e-9]
  Three-Phase Series RLC Branch : spsThreePhaseSeriesRLCBranchLib/Three-Phase Series RLC Branch  LConnTagsString=A|B|C  RConnTagsString=A|B|C  BranchType=RL  Resistance=1  Inductance=1e-3  Capacitance=1e-6  Measurements=None
  Three-Phase Series RLC Branch1 : spsThreePhaseSeriesRLCBranchLib/Three-Phase Series RLC Branch  LConnTagsString=A|B|C  RConnTagsString=A|B|C  BranchType=L  Resistance=1  Inductance=4e-3  Capacitance=1e-6  Measurements=None
  Three-Phase Transformer (Two Windings){9..10,12,16} (4 alike) : spsThreePhaseTransformerTwoWindingsLib/Three-Phase Transformer (Two Windings)  Winding1Connection=Delta (D11)  Winding2Connection=Yn  CoreType=Three single-phase transformers  SetSaturation=off  Hysteresis=off  DataFile='hysteresis'  SetInitialFlux=off  Measurements=None  UNITS=pu  NominalPower=[ 200000 , 50 ]  Winding1=[ 11e3 , 0.002 , 0.08 ]  Winding2=[ 0.23e3 , 0.002 , 0.08 ]  Rm=500  Lm=500  L0=0.5  Saturation=[ 0,0 ; 0.0024,1.2 ; 1.0,1.52 ]  InitialFluxes=[ 0.8 , -0.8 , 0.7 ]  BreakLoop=off  DiscreteSolver=Trapezoidal iterative  DataType=off  TransfoNumber=1
  Three-Phase Fault{,1..3} (4 alike) : spsThreePhaseFaultLib/Three-Phase Fault  InitialStates=0  FaultA=on  FaultB=on  FaultC=on  GroundFault=on  SwitchTimes="[1  2]"  External=off  SwitchStatus=NaN  FaultResistance=0.001  GroundResistance=0.01  SnubberResistance=1e6  SnubberCapacitance=inf  Measurements=None
  To Workspace : ToWorkspace  VariableName=va  SampleTime=-1
  To Workspace1 : ToWorkspace  VariableName=vb  SampleTime=-1
  To Workspace10 : ToWorkspace  VariableName=ib1  SampleTime=-1
  To Workspace11 : ToWorkspace  VariableName=ic1  SampleTime=-1
  To Workspace12 : ToWorkspace  VariableName=ib2  SampleTime=-1
  To Workspace13 : ToWorkspace  VariableName=ic2  SampleTime=-1
  To Workspace14 : ToWorkspace  VariableName=va2  SampleTime=-1
  To Workspace15 : ToWorkspace  VariableName=vb2  SampleTime=-1
  To Workspace16 : ToWorkspace  VariableName=vc2  SampleTime=-1
  To Workspace17 : ToWorkspace  VariableName=ia2  SampleTime=-1
  To Workspace18 : ToWorkspace  VariableName=ib3  SampleTime=-1
  To Workspace19 : ToWorkspace  VariableName=ic3  SampleTime=-1
  To Workspace2 : ToWorkspace  VariableName=vc  SampleTime=-1
  To Workspace20 : ToWorkspace  VariableName=va3  SampleTime=-1
  To Workspace21 : ToWorkspace  VariableName=vb3  SampleTime=-1
  To Workspace22 : ToWorkspace  VariableName=vc3  SampleTime=-1
  To Workspace23 : ToWorkspace  VariableName=ia3  SampleTime=-1
  To Workspace3 : ToWorkspace  VariableName=ia  SampleTime=-1
  To Workspace4 : ToWorkspace  VariableName=ib  SampleTime=-1
  To Workspace5 : ToWorkspace  VariableName=ic  SampleTime=-1
  To Workspace6 : ToWorkspace  VariableName=va1  SampleTime=-1
  To Workspace7 : ToWorkspace  VariableName=vb1  SampleTime=-1
  To Workspace8 : ToWorkspace  VariableName=vc1  SampleTime=-1
  To Workspace9 : ToWorkspace  VariableName=ia1  SampleTime=-1
  Voltage{,1..3} (4 alike) : Demux  Outputs=3
  _ : spsThreePhaseTransformerTwoWindingsLib/Three-Phase Transformer (Two Windings)  Winding1Connection=Delta (D11)  Winding2Connection=Yn  CoreType=Three single-phase transformers  SetSaturation=off  Hysteresis=off  DataFile='hysteresis'  SetInitialFlux=off  Measurements=None  UNITS=pu  NominalPower=[ 100000 , 50 ]  Winding1=[11e3 , 0.002 , 0.08 ]  Winding2=[ 0.23e3 , 0.002 , 0.08 ]  Rm=500  Lm=500  L0=0.5  Saturation=[ 0,0 ; 0.0024,1.2 ; 1.0,1.52 ]  InitialFluxes=[ 0.8 , -0.8 , 0.7 ]  BreakLoop=off  DiscreteSolver=Trapezoidal iterative  DataType=off  TransfoNumber=1
  __ : spsThreePhaseTransformerTwoWindingsLib/Three-Phase Transformer (Two Windings)  Winding1Connection=Delta (D11)  Winding2Connection=Yn  CoreType=Three single-phase transformers  SetSaturation=off  Hysteresis=off  DataFile='hysteresis'  SetInitialFlux=off  Measurements=None  UNITS=pu  NominalPower=[ 300000 , 50 ]  Winding1=[11e3 , 0.002 , 0.08 ]  Winding2=[ 0.23e3 , 0.002 , 0.08 ]  Rm=500  Lm=500  L0=0.5  Saturation=[ 0,0 ; 0.0024,1.2 ; 1.0,1.52 ]  InitialFluxes=[ 0.8 , -0.8 , 0.7 ]  BreakLoop=off  DiscreteSolver=Trapezoidal iterative  DataType=off  TransfoNumber=1
  powergui : spspowerguiLib/powergui  Priority=1  SimulationMode=Discrete  SampleTime=50e-6  frequency=50  Iterations=50  frequencyindice=50  Pbase=100e6  ErrMax=1e-4  UnitsV=kV  UnitsW=MW  buscounter=43  FunctionMessages=off  echomessages=off  EnableUseOfTLC=off  CurrentSourceSwitches=off  DisableSnubberDevices=off  DisableRonSwitches=off  DisableVfSwitches=off  DisplayEquations=off  AutomaticDiscreteSolvers=off  SolverType=Tustin/Backward Euler (TBE)  Interpol=off  ExternalGateDelay=off  methode=off  Ts=100  x0status=blocks  SPID=on  SwTol=0  HookPort=off  NonlinearTolerance=1e-4  nMaxIteration=100  ContinueOnMaxIteration=off  RestoreLinks=warning  ResistiveCurrentMeasurement=off  Frange=[0:2:500]  Ylog=off  Xlog=on  ShowGrid=off  save=off  variable=ZData  structure=0  ZoomFFT=off  StartTime=0.0  cycles=1  DisplayStyle=1  fundamental=60  FreqAxis=off  MaxFrequency=1000  frequencyindicesteady=1  RmsSteady=1  display=off
  thapathali switching : spsThreePhaseSourceLib/Three-Phase Source  InternalConnection=Yg  VoltagePhases=off  Voltage=(11000)*1.00021  PhaseAngle=0.019125  Voltage_phases=[11e3 11e3 11e3]/sqrt(3)  PhaseAngles_phases=[0 -120 +120]  Frequency=50  NonIdealSource=on  SpecifyImpedance=off  Resistance=0.8929  Inductance=16.58e-3  ShortCircuitLevel=100e6  BaseVoltage=11e3  XRratio=7  BusType=swing  Pref=10000  Qref=0  Prefabc=[10e3, 10e3, 10e3]  Qrefabc=[0, 0, 0]  Qmin=-Inf  Qmax=Inf
  wires:
  1/1 -> Voltage/1
  1/2 -> Current/1
  Voltage/1 -> To Workspace/1
  Voltage/2 -> To Workspace1/1
  Voltage/3 -> To Workspace2/1
  Current/2 -> To Workspace4/1
  Current/1 -> To Workspace3/1
  Current/3 -> To Workspace5/1
  0/1 -> Voltage1/1
  Voltage1/1 -> To Workspace6/1
  Current1/1 -> To Workspace9/1
  Current1/3 -> To Workspace11/1
  Voltage1/2 -> To Workspace7/1
  0/2 -> Current1/1
  Voltage1/3 -> To Workspace8/1
  Current1/2 -> To Workspace10/1
  Current2/3 -> To Workspace13/1
  3/1 -> Voltage2/1
  Current2/1 -> To Workspace17/1
  Current2/2 -> To Workspace12/1
  Voltage2/1 -> To Workspace14/1
  3/2 -> Current2/1
  Voltage2/3 -> To Workspace16/1
  Voltage2/2 -> To Workspace15/1
  Voltage3/1 -> To Workspace20/1
  Current3/1 -> To Workspace23/1
  Current3/2 -> To Workspace18/1
  Voltage3/2 -> To Workspace21/1
  Voltage3/3 -> To Workspace22/1
  Current3/3 -> To Workspace19/1
  2/1 -> Voltage3/1
  2/2 -> Current3/1
  connections:
  Three-Phase Transformer (Two Windings)12/LConn1 -- Three-Phase PI Section Line5/RConn1 -- Sajha 500KVA/LConn1 -- Bus*35*/LConn1 -- Three-Phase PI Section Line14/LConn1 -- Three-Phase PI Section Line13/RConn1
  Three-Phase PI Section Line3/RConn3 -- Three-Phase PI Section Line4/LConn3 -- Salik Chwok 200KVA/LConn3
  Three-Phase Transformer (Two Windings)16/LConn3 -- Three-Phase PI Section Line12/LConn3 -- Three-Phase Fault3/LConn3 -- 2/RConn3
  Kandebata Sthan 300KVA/LConn1 -- Bus*30*/LConn1 -- Three-Phase PI Section Line17/RConn1 -- Three-Phase PI Section Line/RConn1 -- Three-Phase Series RLC Branch/LConn1 -- Three-Phase PI Section Line1/LConn1
  Pulchwok Campus Wall 200KVA/LConn2 -- Three-Phase PI Section Line4/RConn2 -- Three-Phase PI Section Line7/LConn2
  Bima Samiti 200KVA/LConn2 -- Three-Phase PI Section Line17/LConn2 -- Sarbanga Hospital 200KVA/LConn2
  Three-Phase PI Section Line1/RConn1 -- _/LConn1 -- Bus*41*/LConn1 -- Three-Phase PI Section Line2/LConn1
  Three-Phase PI Section Line7/RConn2 -- Three-Phase Fault2/LConn2 -- 3/RConn2 -- Three-Phase PI Section Line5/LConn2 -- .../LConn2 -- Three-Phase PI Section Line18/LConn2 -- Bakhundol Mode 300KVA/LConn2
  Three-Phase PI Section Line9/LConn1 -- Three-Phase PI Section Line8/RConn1 -- Bakhundol Kutumba Hotel 200KVA/LConn1 -- Bus*29*/LConn1
  Three-Phase Transformer (Two Windings)10/LConn3 -- Three-Phase PI Section Line15/RConn3 -- Three-Phase PI Section Line16/LConn3
  Three-Phase PI Section Line5/RConn3 -- Sajha 500KVA/LConn3 -- Three-Phase Transformer (Two Windings)12/LConn3 -- Three-Phase PI Section Line13/RConn3 -- Three-Phase PI Section Line14/LConn3
  Three-Phase PI Section Line8/LConn3 -- Bakhundol Carwash 200KVA/LConn3 -- Three-Phase PI Section Line18/RConn3
  Three-Phase Transformer (Two Windings)10/LConn2 -- Three-Phase PI Section Line15/RConn2 -- Three-Phase PI Section Line16/LConn2
  Three-Phase Transformer (Two Windings)16/LConn2 -- Three-Phase PI Section Line12/LConn2 -- Three-Phase Fault3/LConn2 -- 2/RConn2
  Three-Phase PI Section Line14/LConn2 -- Three-Phase Transformer (Two Windings)12/LConn2 -- Three-Phase PI Section Line13/RConn2 -- Sajha 500KVA/LConn2 -- Three-Phase PI Section Line5/RConn2
  .../LConn3 -- Three-Phase Fault2/LConn3 -- 3/RConn3 -- Three-Phase PI Section Line18/LConn3 -- Bakhundol Mode 300KVA/LConn3 -- Three-Phase PI Section Line7/RConn3 -- Three-Phase PI Section Line5/LConn3
  Three-Phase PI Section Line8/LConn1 -- Three-Phase PI Section Line18/RConn1 -- Bakhundol Carwash 200KVA/LConn1 -- Bus*27*/LConn1
  Three-Phase PI Section Line8/RConn3 -- Three-Phase PI Section Line9/LConn3 -- Bakhundol Kutumba Hotel 200KVA/LConn3
  Three-Phase PI Section Line14/RConn2 -- Three-Phase Transformer (Two Windings)9/LConn2 -- Three-Phase PI Section Line15/LConn2
  Three-Phase PI Section Line7/RConn1 -- Three-Phase Fault2/LConn1 -- 3/RConn1 -- Bus*24*/LConn1 -- .../LConn1 -- Three-Phase PI Section Line5/LConn1 -- Three-Phase PI Section Line18/LConn1 -- Bakhundol Mode 300KVA/LConn1 -- Bus*25*/LConn1
  _/LConn2 -- Three-Phase PI Section Line2/LConn2 -- Three-Phase PI Section Line1/RConn2
  Three-Phase PI Section Line11/LConn1 -- High Court 200KVA/LConn1 -- Bus*37*/LConn1 -- 2/LConn1 -- Three-Phase PI Section Line10/RConn1
  Three-Phase PI Section Line2/RConn3 -- Three-Phase PI Section Line3/LConn3 -- __/LConn3
  Three-Phase PI Section Line2/RConn1 -- Three-Phase PI Section Line3/LConn1 -- __/LConn1 -- Bus*43*/LConn1
  Three-Phase PI Section Line1/LConn3 -- Three-Phase PI Section Line17/RConn3 -- Kandebata Sthan 300KVA/LConn3 -- Three-Phase PI Section Line/RConn3 -- Three-Phase Series RLC Branch/LConn3
  Bakhundol Carwash 200KVA/LConn2 -- Three-Phase PI Section Line18/RConn2 -- Three-Phase PI Section Line8/LConn2
  _/LConn3 -- Three-Phase PI Section Line2/LConn3 -- Three-Phase PI Section Line1/RConn3
  Three-Phase PI Section Line4/RConn1 -- Three-Phase PI Section Line7/LConn1 -- Pulchwok Campus Wall 200KVA/LConn1 -- Bus*26*/LConn1
  Three-Phase PI Section Line3/RConn2 -- Three-Phase PI Section Line4/LConn2 -- Salik Chwok 200KVA/LConn2
  Bima Samiti 200KVA/LConn3 -- Three-Phase PI Section Line17/LConn3 -- Sarbanga Hospital 200KVA/LConn3
  Three-Phase PI Section Line16/LConn1 -- Three-Phase PI Section Line15/RConn1 -- Three-Phase Transformer (Two Windings)10/LConn1 -- Bus*33*/LConn1
  Three-Phase PI Section Line/RConn2 -- Three-Phase Series RLC Branch/LConn2 -- Three-Phase PI Section Line1/LConn2 -- Three-Phase PI Section Line17/RConn2 -- Kandebata Sthan 300KVA/LConn2
  Three-Phase PI Section Line2/RConn2 -- Three-Phase PI Section Line3/LConn2 -- __/LConn2
  Three-Phase PI Section Line4/RConn3 -- Three-Phase PI Section Line7/LConn3 -- Pulchwok Campus Wall 200KVA/LConn3
  Three-Phase PI Section Line14/RConn3 -- Three-Phase Transformer (Two Windings)9/LConn3 -- Three-Phase PI Section Line15/LConn3
  Three-Phase PI Section Line8/RConn2 -- Bakhundol Kutumba Hotel 200KVA/LConn2 -- Three-Phase PI Section Line9/LConn2
  Three-Phase PI Section Line3/RConn1 -- Three-Phase PI Section Line4/LConn1 -- Salik Chwok 200KVA/LConn1 -- Bus*23*/LConn1
  Sarbanga Hospital 200KVA/LConn1 -- Three-Phase PI Section Line17/LConn1 -- Bima Samiti 200KVA/LConn1 -- Bus*22*/LConn1
  Three-Phase PI Section Line14/RConn1 -- Three-Phase Transformer (Two Windings)9/LConn1 -- Bus*39*/LConn1 -- Three-Phase PI Section Line15/LConn1
  Three-Phase PI Section Line9/RConn2 -- Sarwanga Hospital 300KVA/LConn2
  Three-Phase Transformer (Two Windings)12/RConn1 -- Bus*34*/LConn1 -- Norvic Hospital Load/LConn1
  Three-Phase PI Section Line11/RConn2 -- Pariwar Niyojan 100KVA/LConn2
  ../RConn1 -- Labim Mall Load/LConn1 -- Bus*12*/LConn1
  Three-Phase PI Section Line9/RConn3 -- Sarwanga Hospital 300KVA/LConn3
  Sarwanga Hospital 300KVA/RConn1 -- Sarwanga Hospital Load/LConn1 -- Bus*8*/LConn1
  Three-Phase PI Section Line16/RConn2 -- ../LConn2
  Sarbanga Hospital 200KVA/RConn1 -- Sarbanga Hospital Load/LConn1 -- Bus*17*/LConn1
  Three-Phase PI Section Line13/LConn1 -- NEA Charging Station/LConn1 -- Bus*20*/LConn1
  Three-Phase Transformer (Two Windings)9/RConn1 -- Manab Adhikar Office Inside Load/LConn1 -- Bus*38*/LConn1
  Bus*4*/LConn1 -- Bakhundol Mode Load/LConn1 -- Bakhundol Mode 300KVA/RConn1
  _/RConn3 -- Jwagal Chowk Load/LConn3
  Three-Phase PI Section Line11/RConn1 -- Pariwar Niyojan 100KVA/LConn1 -- Bus*18*/LConn1
  Salik Chwok 200KVA/RConn1 -- Salik Chowk Load/LConn1 -- Bus*2*/LConn1
  Jall Utpanna Office 100KVA/RConn1 -- Jal Utpanna Office Load/LConn1 -- Bus*16*/LConn1
  Three-Phase PI Section Line12/RConn3 -- Jall Utpanna Office 100KVA/LConn3
  Bus*14*/LConn1 -- HIgh Court Load/LConn1 -- High Court 200KVA/RConn1
  NEA Charging Station/RConn1 -- NEA Charging Station Load/LConn1 -- Bus*11*/LConn1
  Three-Phase PI Section Line12/RConn2 -- Jall Utpanna Office 100KVA/LConn2
  Three-Phase PI Section Line16/RConn3 -- ../LConn3
  _/RConn2 -- Jwagal Chowk Load/LConn2
  Three-Phase Transformer (Two Windings)10/RConn1 -- Manab Adhikar Wall Load/LConn1 -- Bus*32*/LConn1
  Pulchwok Campus Wall 200KVA/RConn1 -- Pulchowk Campus Load/LConn1 -- Bus*3*/LConn1
  Bakhundol Carwash 200KVA/RConn1 -- Bakhundol Car Wash Load/LConn1 -- Bus*5*/LConn1
  .../RConn1 -- Bus*7*/LConn1 -- NTC Office Load/LConn1
  NEA Charging Station/LConn3 -- Three-Phase PI Section Line13/LConn3
  Sarwanga Hospital 300KVA/LConn1 -- Three-Phase PI Section Line9/RConn1 -- Bus*28*/LConn1
  _/RConn1 -- Jwagal Chowk Load/LConn1 -- Bus*40*/LConn1
  Bima Samiti 200KVA/RConn1 -- Bima Samiti Load/LConn1 -- Bus*10*/LConn1
  __/RConn1 -- HImalaya Hotel Load/LConn1 -- Bus*42*/LConn1
  Bakhundol Kutumba Hotel 200KVA/RConn1 -- Bakhundol Kutumba Hotel Load/LConn1 -- Bus*6*/LConn1
  NEA Charging Station/LConn2 -- Three-Phase PI Section Line13/LConn2
  Pariwar Niyojan 100KVA/RConn1 -- Pariwar Niyojan Load/LConn1 -- Bus*15*/LConn1
  Kandebata Sthan 300KVA/RConn1 -- Kandevatasthan Load/LConn1 -- Bus*9*/LConn1
  Jall Utpanna Office 100KVA/LConn1 -- Three-Phase PI Section Line12/RConn1 -- Bus*19*/LConn1
  Bus*36*/LConn1 -- Jal Utpanna Office Wall Side Load/LConn1 -- Three-Phase Transformer (Two Windings)16/RConn1
  Pariwar Niyojan 100KVA/LConn3 -- Three-Phase PI Section Line11/RConn3
  ../LConn1 -- Three-Phase PI Section Line16/RConn1 -- Bus*21*/LConn1
  Sajha 500KVA/RConn1 -- Sajha Load/LConn1 -- Bus*1*/LConn1
  0/LConn1 -- Three-Phase Series RLC Branch/RConn1
  0/LConn2 -- Three-Phase Series RLC Branch/RConn2
  0/LConn3 -- Three-Phase Series RLC Branch/RConn3
  0/RConn1 -- Three-Phase Fault1/LConn1 -- Three-Phase Series RLC Branch1/LConn1
  0/RConn2 -- Three-Phase Series RLC Branch1/LConn2 -- Three-Phase Fault1/LConn2
  0/RConn3 -- Three-Phase Fault1/LConn3 -- Three-Phase Series RLC Branch1/LConn3
  Three-Phase Series RLC Branch1/RConn1 -- ./LConn1 -- Bus*31*/LConn1
  ./LConn2 -- Three-Phase Series RLC Branch1/RConn2
  ./LConn3 -- Three-Phase Series RLC Branch1/RConn3
  Kandevatasthan Opposite Load/LConn1 -- ./RConn1 -- Bus*13*/LConn1
  thapathali switching/RConn1 -- Load Flow Bus/LConn1 -- 1/LConn1
  thapathali switching/RConn2 -- 1/LConn2
  thapathali switching/RConn3 -- 1/LConn3
  1/RConn1 -- Three-Phase Fault/LConn1 -- Three-Phase PI Section Line/LConn1
  1/RConn2 -- Three-Phase Fault/LConn2 -- Three-Phase PI Section Line/LConn2
  1/RConn3 -- Three-Phase Fault/LConn3 -- Three-Phase PI Section Line/LConn3
  Kandevatasthan Opposite Load/LConn2 -- ./RConn2
  Kandevatasthan Opposite Load/LConn3 -- ./RConn3
  Kandebata Sthan 300KVA/RConn2 -- Kandevatasthan Load/LConn2
  Kandebata Sthan 300KVA/RConn3 -- Kandevatasthan Load/LConn3
  Kandebata Sthan 300KVA/RConn4 -- Kandevatasthan Load/RConn1
  Jwagal Chowk Load/RConn1 -- _/RConn4
  HImalaya Hotel Load/LConn2 -- __/RConn2
  __/RConn3 -- HImalaya Hotel Load/LConn3
  __/RConn4 -- HImalaya Hotel Load/RConn1
  Salik Chwok 200KVA/RConn4 -- Salik Chowk Load/RConn1
  Salik Chowk Load/LConn2 -- Salik Chwok 200KVA/RConn2
  Salik Chwok 200KVA/RConn3 -- Salik Chowk Load/LConn3
  Pulchowk Campus Load/LConn2 -- Pulchwok Campus Wall 200KVA/RConn2
  Pulchowk Campus Load/LConn3 -- Pulchwok Campus Wall 200KVA/RConn3
  Pulchowk Campus Load/RConn1 -- Pulchwok Campus Wall 200KVA/RConn4
  NTC Office Load/LConn2 -- .../RConn2
  NTC Office Load/LConn3 -- .../RConn3
  NTC Office Load/RConn1 -- .../RConn4
  Sajha Load/LConn2 -- Sajha 500KVA/RConn2
  Sajha Load/LConn3 -- Sajha 500KVA/RConn3
  Sajha Load/RConn1 -- Sajha 500KVA/RConn4
  NEA Charging Station Load/LConn2 -- NEA Charging Station/RConn2
  NEA Charging Station Load/LConn3 -- NEA Charging Station/RConn3
  NEA Charging Station Load/RConn1 -- NEA Charging Station/RConn4
  Norvic Hospital Load/LConn2 -- Three-Phase Transformer (Two Windings)12/RConn2
  Norvic Hospital Load/LConn3 -- Three-Phase Transformer (Two Windings)12/RConn3
  Norvic Hospital Load/RConn1 -- Three-Phase Transformer (Two Windings)12/RConn4
  Manab Adhikar Office Inside Load/LConn2 -- Three-Phase Transformer (Two Windings)9/RConn2
  Manab Adhikar Office Inside Load/LConn3 -- Three-Phase Transformer (Two Windings)9/RConn3
  Three-Phase Transformer (Two Windings)9/RConn4 -- Manab Adhikar Office Inside Load/RConn1
  Manab Adhikar Wall Load/LConn2 -- Three-Phase Transformer (Two Windings)10/RConn2
  Manab Adhikar Wall Load/LConn3 -- Three-Phase Transformer (Two Windings)10/RConn3
  Manab Adhikar Wall Load/RConn1 -- Three-Phase Transformer (Two Windings)10/RConn4
  Labim Mall Load/LConn2 -- ../RConn2
  Labim Mall Load/LConn3 -- ../RConn3
  ../RConn4 -- Labim Mall Load/RConn1
  Bakhundol Mode 300KVA/RConn2 -- Bakhundol Mode Load/LConn2
  Bakhundol Mode 300KVA/RConn3 -- Bakhundol Mode Load/LConn3
  Bakhundol Mode 300KVA/RConn4 -- Bakhundol Mode Load/RConn1
  Bakhundol Car Wash Load/LConn2 -- Bakhundol Carwash 200KVA/RConn2
  Bakhundol Car Wash Load/LConn3 -- Bakhundol Carwash 200KVA/RConn3
  Bakhundol Carwash 200KVA/RConn4 -- Bakhundol Car Wash Load/RConn1
  Bakhundol Kutumba Hotel Load/LConn2 -- Bakhundol Kutumba Hotel 200KVA/RConn2
  Bakhundol Kutumba Hotel Load/LConn3 -- Bakhundol Kutumba Hotel 200KVA/RConn3
  Bakhundol Kutumba Hotel 200KVA/RConn4 -- Bakhundol Kutumba Hotel Load/RConn1
  Sarwanga Hospital Load/LConn2 -- Sarwanga Hospital 300KVA/RConn2
  Sarwanga Hospital Load/LConn3 -- Sarwanga Hospital 300KVA/RConn3
  Sarwanga Hospital 300KVA/RConn4 -- Sarwanga Hospital Load/RConn1
  HIgh Court Load/LConn2 -- High Court 200KVA/RConn2
  HIgh Court Load/LConn3 -- High Court 200KVA/RConn3
  High Court 200KVA/RConn4 -- HIgh Court Load/RConn1
  Pariwar Niyojan Load/LConn2 -- Pariwar Niyojan 100KVA/RConn2
  Pariwar Niyojan Load/LConn3 -- Pariwar Niyojan 100KVA/RConn3
  Pariwar Niyojan 100KVA/RConn4 -- Pariwar Niyojan Load/RConn1
  Jal Utpanna Office Load/LConn2 -- Jall Utpanna Office 100KVA/RConn2
  Jal Utpanna Office Load/LConn3 -- Jall Utpanna Office 100KVA/RConn3
  Jall Utpanna Office 100KVA/RConn4 -- Jal Utpanna Office Load/RConn1
  Jal Utpanna Office Wall Side Load/LConn2 -- Three-Phase Transformer (Two Windings)16/RConn2
  Jal Utpanna Office Wall Side Load/LConn3 -- Three-Phase Transformer (Two Windings)16/RConn3
  Three-Phase Transformer (Two Windings)16/RConn4 -- Jal Utpanna Office Wall Side Load/RConn1
  Bima Samiti Load/LConn2 -- Bima Samiti 200KVA/RConn2
  Bima Samiti Load/LConn3 -- Bima Samiti 200KVA/RConn3
  Bima Samiti 200KVA/RConn4 -- Bima Samiti Load/RConn1
  Sarbanga Hospital Load/LConn2 -- Sarbanga Hospital 200KVA/RConn2
  Sarbanga Hospital Load/LConn3 -- Sarbanga Hospital 200KVA/RConn3
  Sarbanga Hospital 200KVA/RConn4 -- Sarbanga Hospital Load/RConn1
  Three-Phase Transformer (Two Windings)16/LConn1 -- Three-Phase PI Section Line12/LConn1 -- Three-Phase Fault3/LConn1 -- 2/RConn1
  Three-Phase PI Section Line10/RConn2 -- 2/LConn2 -- Three-Phase PI Section Line11/LConn2 -- High Court 200KVA/LConn2
  Three-Phase PI Section Line11/LConn3 -- High Court 200KVA/LConn3 -- Three-Phase PI Section Line10/RConn3 -- 2/LConn3
  3/LConn1 -- Three-Phase PI Section Line10/LConn1
  Three-Phase PI Section Line10/LConn3 -- 3/LConn3
  3/LConn2 -- Three-Phase PI Section Line10/LConn2
